simulink model "dc_converter"  (R2024a)
settings: Solver=VariableStepAuto  StartTime=0.0  StopTime=20  RelTol=1e-3
libraries: simulink x2
settings Model: Creator=emanuele  LastModifiedBy=emanuele

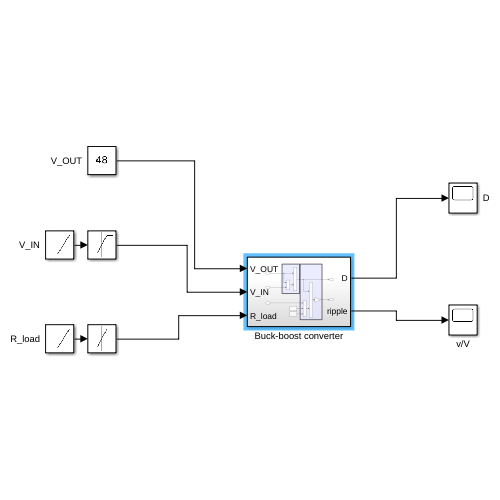
[thumbnail: Simulink's stored preview of the top-level diagram]
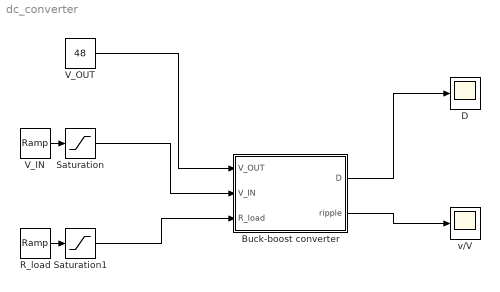
== system dc_converter ==
  Buck-boost converter : Subsystem
  D : Scope
  R_load : simulink/Sources/Ramp  slope=-1  start=10  InitialOutput=5
  Saturation : Saturate  UpperLimit=160  LowerLimit=24
  Saturation1 : Saturate  UpperLimit=5  LowerLimit=1
  V_IN : simulink/Sources/Ramp  slope=-10  start=4  InitialOutput=140
  V_OUT : Constant  Value=48
  v/V : Scope
  wires:
  V_IN/1 -> Saturation/1
  R_load/1 -> Saturation1/1
  V_OUT/1 -> Buck-boost converter/1(V_OUT)
  Saturation/1 -> Buck-boost converter/2(V_IN)
  Saturation1/1 -> Buck-boost converter/3(R_load)
  Buck-boost converter/1(D) -> D/1
  Buck-boost converter/2(ripple) -> v/V/1

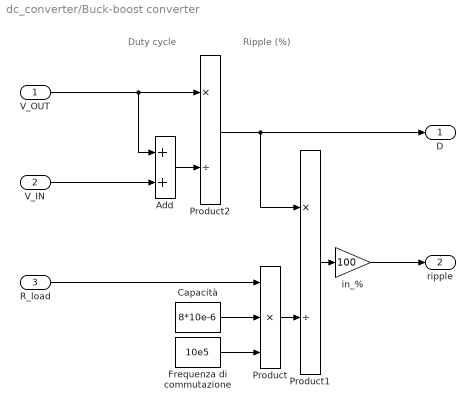
== system dc_converter/Buck-boost converter ==
  note: Duty cycle
  note: Ripple (%)
  V_OUT : Inport  Unit=V
  V_IN : Inport  Port=2  Unit=V
  R_load : Inport  Port=3  Unit=Ω
  Add : Sum
  Capacità : Constant  Value=8*10e-6
  Frequenza di commutazione : Constant  Value=10e5
  Product : Product  Inputs=3
  Product1 : Product  Inputs=*/
  Product2 : Product  Inputs=*/
  in_% : Gain  Gain=100
  D : Outport  Unit=1
  ripple : Outport  Port=2  Unit=%
  wires:
  R_load/1 -> Product/1
  Capacità/1 -> Product/2
  V_IN/1 -> Add/2
  Frequenza di commutazione/1 -> Product/3
  Product/1 -> Product1/2
  V_OUT/1 -> Product2/1, Add/1
  Add/1 -> Product2/2
  Product1/1 -> in_%/1
  in_%/1 -> ripple/1
  Product2/1 -> D/1, Product1/1
